simulink model "innerControllerTuning3"  (R2018a)
settings: Solver=VariableStepAuto  StartTime=0.0  StopTime=60  RelTol=1e-3
values from neighbouring files (symbols this model uses):
  d = 2.4*10^-3    (= 0.0024)    [innerInit.m]    (also in outerInit.m)
  dx0 = 0    [innerInit.m]
  dy0 = 0    [innerInit.m]
  dz0 = 0    [innerInit.m]
  g = 9.81    [innerInit.m]    (also in outerInit.m)
  Ixx = 5.9*10-3    (= 56)    [innerInit.m]    (also in outerInit.m = 0.0059)
  Iyy = 5.9*10-3    (= 56)    [innerInit.m]    (also in outerInit.m = 0.0059)
  Izz = 1.16*10-3    (= 8.6)    [innerInit.m]    (also in outerInit.m = 0.00116)
  K_lin = [   15.6000,    0.0000,    7.9000,    0.0000,         0 ... (first row only)    [innerInit.m]
  kr = 0.1    [innerInit.m]    (also in outerInit.m)
  kt = 0.1    [innerInit.m]    (also in outerInit.m)
  l = 0.255    [innerInit.m]    (also in outerInit.m)
  m = 0.5    [innerInit.m]    (also in outerInit.m)
  p0 = 0.5    [innerInit.m]
  phi0 = pi/4    (= 0.785398163397)    [innerInit.m]
  psi0 = pi/4    (= 0.785398163397)    [innerInit.m]
  q0 = 0.5    [innerInit.m]
  r0 = 2.7    [innerInit.m]
  theta0 = pi/4    (= 0.785398163397)    [innerInit.m]
  x0 = 1    [innerInit.m]    (also in outerInit.m = 2)
  y0 = 1    [innerInit.m]    (also in outerInit.m = 3)
  z0 = 0    [innerInit.m]    (also in outerInit.m = 4)
libraries: aerolibutil x1
settings Model: Creator=giuseppe  LastModifiedBy=giuseppe

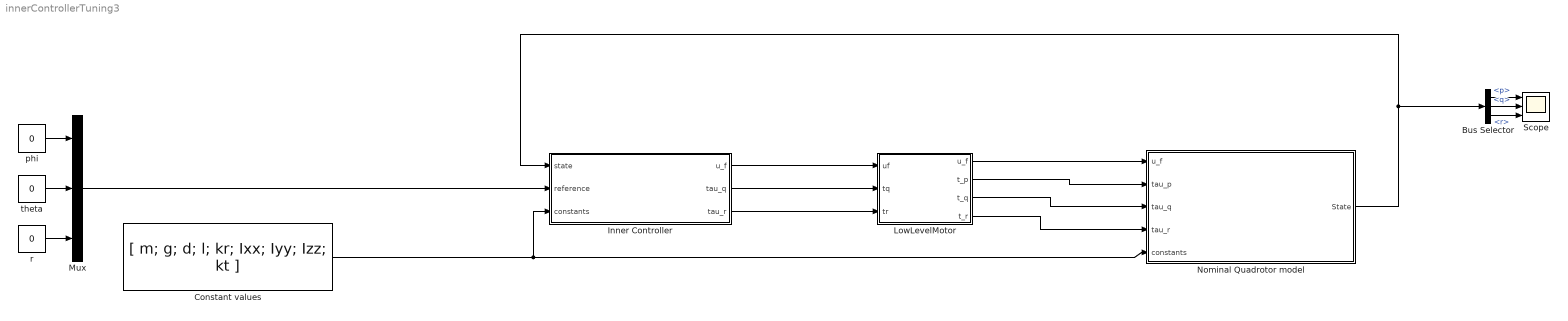
== system innerControllerTuning3 ==
  Bus Selector : BusSelector  OutputSignals=p,q,r
  Constant values : Constant  Value=[ m; g; d; l; kr; Ixx; Iyy; Izz; kt ]
  "Inner Controller " : Subsystem
  LowLevelMotor : Subsystem
  Mux : Mux  Inputs=3
  Nominal Quadrotor model : Subsystem
  Scope : Scope  NumInputPorts=3
  phi : Constant  Value=0
  r : Constant  Value=0
  theta : Constant  Value=0
  wires:
  LowLevelMotor/1(u_f) -> Nominal Quadrotor model/1(u_f)
  "Inner Controller "/2(tau_q) -> LowLevelMotor/2("tq ")
  LowLevelMotor/2(t_p) -> Nominal Quadrotor model/2(tau_p)
  "Inner Controller "/3(tau_r) -> LowLevelMotor/3(tr)
  "Inner Controller "/1(u_f) -> LowLevelMotor/1(uf)
  LowLevelMotor/3(t_q) -> Nominal Quadrotor model/3(tau_q)
  LowLevelMotor/4(t_r) -> Nominal Quadrotor model/4(tau_r)
  Constant values/1 -> "Inner Controller "/3(constants), Nominal Quadrotor model/5(constants)
  Nominal Quadrotor model/1(State) -> Bus Selector/1, "Inner Controller "/1(state)
  Mux/1 -> "Inner Controller "/2(reference)
  phi/1 -> Mux/1
  theta/1 -> Mux/2
  r/1 -> Mux/3
  Bus Selector/1 -> Scope/1  "<p>"
  Bus Selector/2 -> Scope/2  "<q>"
  Bus Selector/3 -> Scope/3  "<r>"

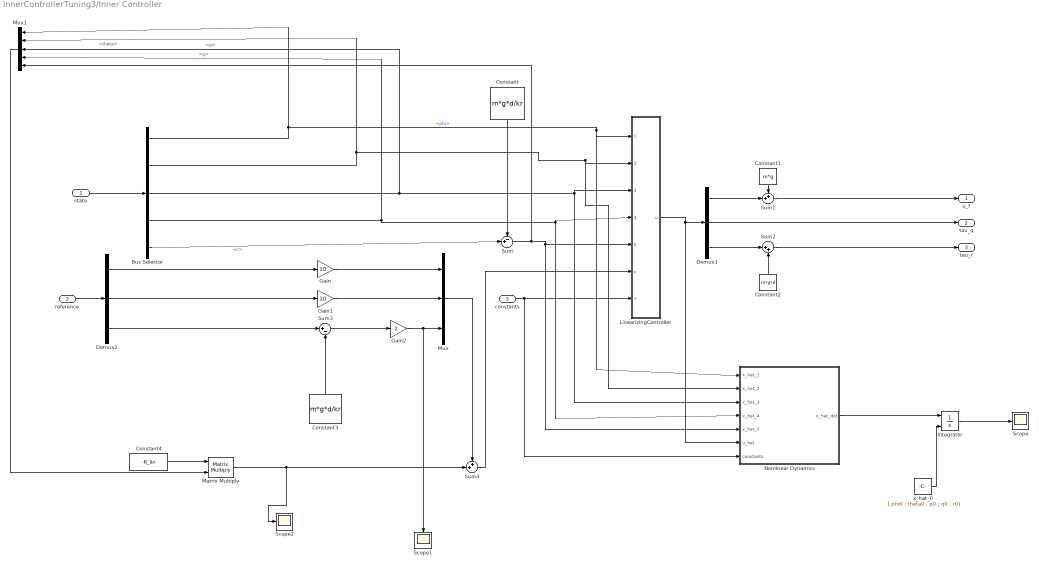
== system innerControllerTuning3/Inner Controller  ==
  state : Inport
  reference : Inport  Port=2
  constants : Inport  Port=3
  Bus Selector : BusSelector  OutputSignals=phi,theta,p,q,r
  Constant : Constant  Value=m*g*d/kr
  Constant1 : Constant  Value=m*g
  Constant2 : Constant  Value=m*g*d
  Constant3 : Constant  Value=m*g*d/kr
  Constant4 : Constant  Value=-K_lin
  Demux1 : Demux  Outputs=3
  Demux2 : Demux  Outputs=3
  Gain : Gain  Gain=10
  Gain1 : Gain  Gain=10
  Gain2 : Gain  Gain=2
  Integrator : Integrator  InitialConditionSource=external
  LinearizingController : MATLAB Function  TreatAsAtomicUnit=on
  Matrix Multiply : Product  Multiplication=Matrix(*)
  Mux : Mux  Inputs=3
  Mux1 : Mux  Inputs=5
  "Nonlinear Dynamics " : MATLAB Function  TreatAsAtomicUnit=on
  Scope : Scope
  Scope1 : Scope
  Scope2 : Scope
  Sum : Sum  Inputs=-+|
  Sum1 : Sum  Inputs=++|
  Sum2 : Sum  Inputs=|++
  Sum3 : Sum  Inputs=|+-
  Sum4 : Sum  Inputs=++|
  x_hat_0 : Constant  Value=[ phi0 ; theta0 ; p0 ; q0 ; r0]
  u_f : Outport
  tau_q : Outport  Port=2
  tau_r : Outport  Port=3
  wires:
  state/1 -> Bus Selector/1
  Bus Selector/3 -> Mux1/3, "Nonlinear Dynamics "/3(x_hat_3), LinearizingController/3(x3_hat)  "<p>"
  Bus Selector/4 -> Mux1/4, "Nonlinear Dynamics "/4(x_hat_4), LinearizingController/4(x4_hat)  "<q>"
  "Nonlinear Dynamics "/1(x_hat_dot) -> Integrator/1
  x_hat_0/1 -> Integrator/2
  Constant/1 -> Sum/1
  Sum/1 -> Mux1/5, "Nonlinear Dynamics "/5(x_hat_5), LinearizingController/5(x5_hat)
  Demux1/3 -> Sum2/1
  Demux1/1 -> Sum1/2
  Constant1/1 -> Sum1/1
  Sum1/1 -> u_f/1
  Demux1/2 -> tau_q/1
  Constant2/1 -> Sum2/2
  Sum2/1 -> tau_r/1
  LinearizingController/1(u) -> "Nonlinear Dynamics "/6(u_hat), Demux1/1
  constants/1 -> "Nonlinear Dynamics "/7(constants), LinearizingController/7(constants)
  Bus Selector/5 -> Sum/2  "<r>"
  reference/1 -> Demux2/1
  Constant3/1 -> Sum3/2
  Sum3/1 -> Gain2/1
  Bus Selector/1 -> Mux1/1, "Nonlinear Dynamics "/1(x_hat_1), LinearizingController/1(x1_hat)  "<phi>"
  Bus Selector/2 -> Mux1/2, "Nonlinear Dynamics "/2(x_hat_2), LinearizingController/2(x2_hat)  "<theta>"
  Demux2/1 -> Gain/1
  Demux2/2 -> Gain1/1
  Constant4/1 -> Matrix Multiply/1
  Mux1/1 -> Matrix Multiply/2
  Mux/1 -> Sum4/1
  Sum4/1 -> LinearizingController/6(v)
  Gain/1 -> Mux/1
  Gain1/1 -> Mux/2
  Demux2/3 -> Sum3/1
  Gain2/1 -> Mux/3, Scope1/1
  Matrix Multiply/1 -> Scope2/1, Sum4/2
  Integrator/1 -> Scope/1

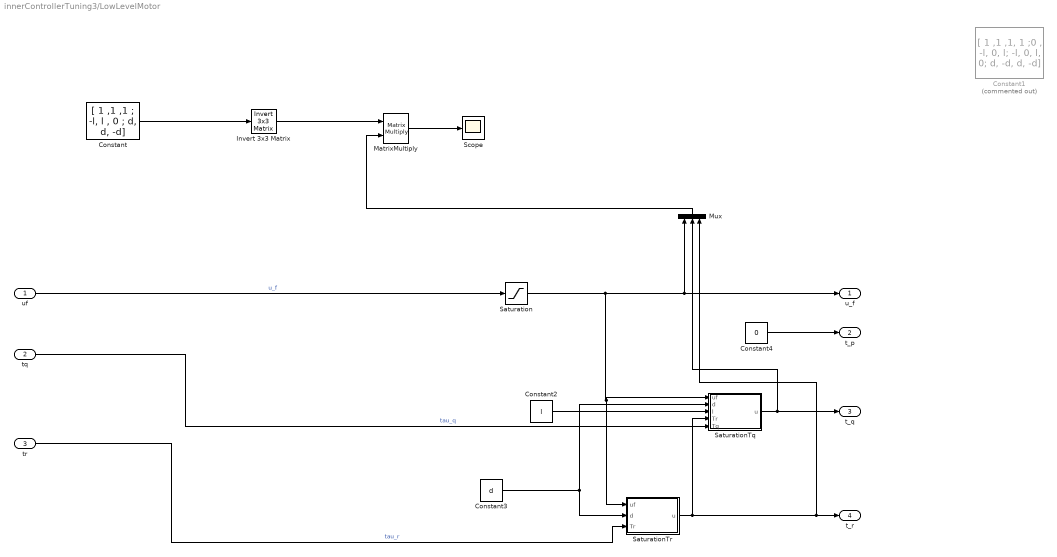
== system innerControllerTuning3/LowLevelMotor ==
  uf : Inport
  "tq " : Inport  Port=2
  tr : Inport  Port=3
  Constant : Constant  Value=[ 1 ,1 ,1 ; -l, l , 0 ; d, d, -d]
  Constant1 : Constant  Commented=on  Value="[ 1 ,1 ,1, 1 ;0 , -l, 0, l;  -l, 0, l, 0; d, -d, d, -d]"
  Constant2 : Constant  Value=l
  Constant3 : Constant  Value=d
  Constant4 : Constant  Value=0
  Invert 3x3 Matrix : aerolibutil/Invert  3x3 Matrix
  MatrixMultiply : Product  Multiplication=Matrix(*)
  Mux : Mux  Inputs=3
  Saturation : Saturate  UpperLimit=30
  SaturationTq : MATLAB Function  TreatAsAtomicUnit=on
  SaturationTr : MATLAB Function  TreatAsAtomicUnit=on
  Scope : Scope
  u_f : Outport
  t_p : Outport  Port=2
  t_q : Outport  Port=3
  t_r : Outport  Port=4
  wires:
  "tq "/1 -> SaturationTq/5(Tq)  "tau_q"
  tr/1 -> SaturationTr/3(Tr)  "tau_r"
  uf/1 -> Saturation/1  "u_f"
  Constant/1 -> Invert 3x3 Matrix/1
  Constant4/1 -> t_p/1
  Constant3/1 -> SaturationTq/2(d), SaturationTr/2(d)
  SaturationTr/1(u) -> SaturationTq/4(Tr), Mux/3, t_r/1
  SaturationTq/1(u) -> Mux/2, t_q/1
  Invert 3x3 Matrix/1 -> MatrixMultiply/1
  Saturation/1 -> SaturationTr/1(uf), SaturationTq/1(uf), u_f/1, Mux/1
  MatrixMultiply/1 -> Scope/1
  Constant2/1 -> SaturationTq/3(l)
  Mux/1 -> MatrixMultiply/2

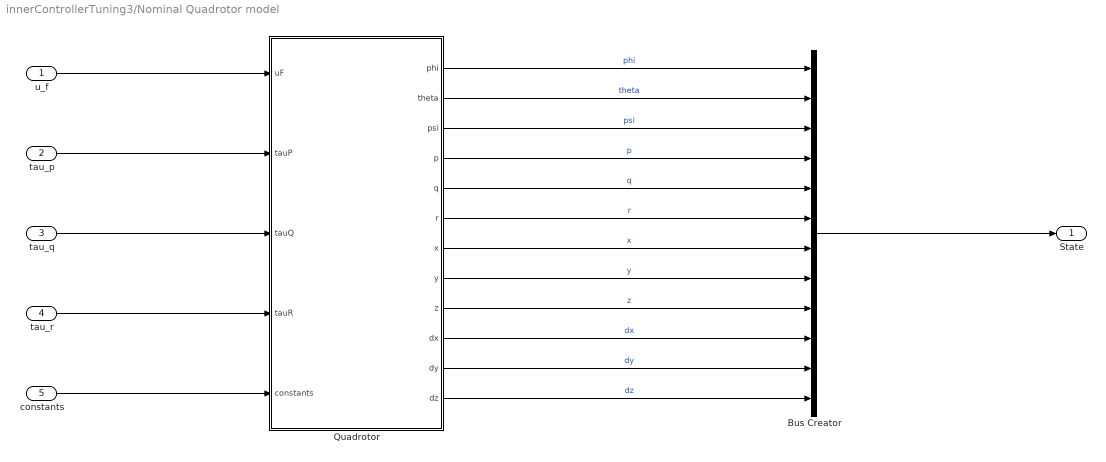
== system innerControllerTuning3/Nominal Quadrotor model ==
  u_f : Inport
  tau_p : Inport  Port=2
  tau_q : Inport  Port=3
  tau_r : Inport  Port=4
  constants : Inport  Port=5
  Bus Creator : BusCreator  Inputs=12
  "Quadrotor " : Subsystem
  State : Outport
  wires:
  u_f/1 -> "Quadrotor "/1(uF)
  tau_q/1 -> "Quadrotor "/3(tauQ)
  tau_r/1 -> "Quadrotor "/4(tauR)
  constants/1 -> "Quadrotor "/5(constants)
  tau_p/1 -> "Quadrotor "/2(tauP)
  "Quadrotor "/1(phi) -> Bus Creator/1  "phi"
  "Quadrotor "/2(theta) -> Bus Creator/2  "theta"
  "Quadrotor "/3(psi) -> Bus Creator/3  "psi"
  "Quadrotor "/4(p) -> Bus Creator/4  "p"
  "Quadrotor "/5(q) -> Bus Creator/5  "q"
  "Quadrotor "/6(r) -> Bus Creator/6  "r"
  "Quadrotor "/7(x) -> Bus Creator/7  "x"
  "Quadrotor "/8(y) -> Bus Creator/8  "y"
  "Quadrotor "/9(z) -> Bus Creator/9  "z"
  Bus Creator/1 -> State/1
  "Quadrotor "/10(dx) -> Bus Creator/10  "dx"
  "Quadrotor "/11(dy) -> Bus Creator/11  "dy"
  "Quadrotor "/12(dz) -> Bus Creator/12  "dz"

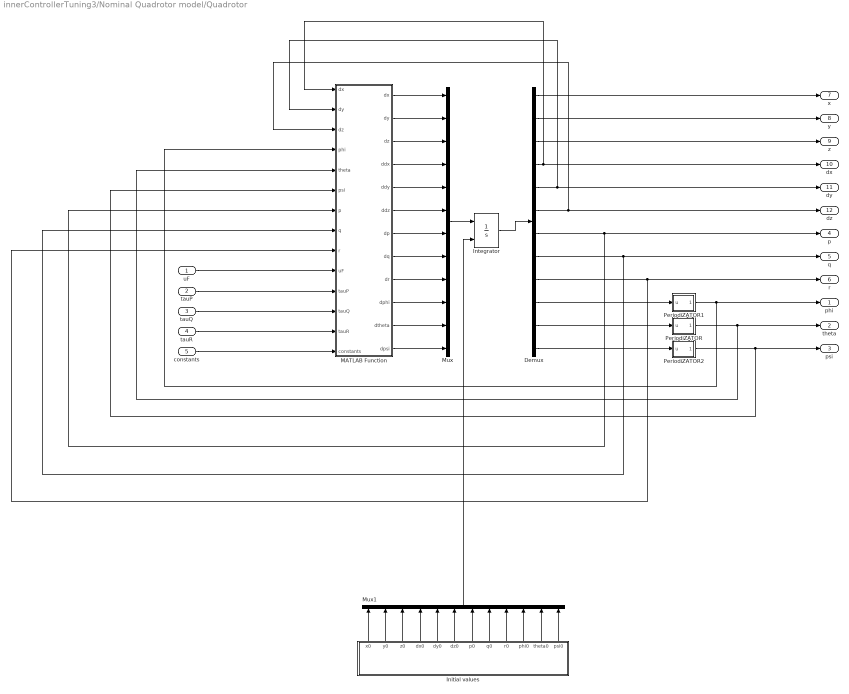
== system innerControllerTuning3/Nominal Quadrotor model/Quadrotor  ==
  uF : Inport
  tauP : Inport  Port=2
  tauQ : Inport  Port=3
  tauR : Inport  Port=4
  constants : Inport  Port=5
  Demux : Demux  Outputs=12
  "Initial values " : Subsystem
  Integrator : Integrator  InitialConditionSource=external
  MATLAB Function : MATLAB Function  TreatAsAtomicUnit=on
  Mux : Mux  Inputs=12
  Mux1 : Mux  Inputs=12
  PeriodiZATOR : MATLAB Function  TreatAsAtomicUnit=on
  PeriodiZATOR1 : MATLAB Function  TreatAsAtomicUnit=on
  PeriodiZATOR2 : MATLAB Function  TreatAsAtomicUnit=on
  phi : Outport
  theta : Outport  Port=2
  psi : Outport  Port=3
  p : Outport  Port=4
  q : Outport  Port=5
  r : Outport  Port=6
  x : Outport  Port=7
  y : Outport  Port=8
  z : Outport  Port=9
  dx : Outport  Port=10
  dy : Outport  Port=11
  dz : Outport  Port=12
  wires:
  uF/1 -> MATLAB Function/10(uF)
  tauP/1 -> MATLAB Function/11(tauP)
  tauQ/1 -> MATLAB Function/12(tauQ)
  tauR/1 -> MATLAB Function/13(tauR)
  PeriodiZATOR/1(angle) -> MATLAB Function/5(theta), theta/1
  PeriodiZATOR1/1(angle) -> MATLAB Function/4(phi), phi/1
  PeriodiZATOR2/1(angle) -> MATLAB Function/6(psi), psi/1
  constants/1 -> MATLAB Function/14(constants)
  MATLAB Function/1(dx) -> Mux/1
  MATLAB Function/2(dy) -> Mux/2
  MATLAB Function/3(dz) -> Mux/3
  MATLAB Function/4(ddx) -> Mux/4
  MATLAB Function/5(ddy) -> Mux/5
  MATLAB Function/6(ddz) -> Mux/6
  MATLAB Function/10(dphi) -> Mux/10
  MATLAB Function/11(dtheta) -> Mux/11
  MATLAB Function/12(dpsi) -> Mux/12
  Mux/1 -> Integrator/1
  "Initial values "/1(x0) -> Mux1/1
  "Initial values "/2(y0) -> Mux1/2
  "Initial values "/3(z0) -> Mux1/3
  "Initial values "/4(dx0) -> Mux1/4
  "Initial values "/5(dy0) -> Mux1/5
  "Initial values "/6(dz0) -> Mux1/6
  "Initial values "/7(p0) -> Mux1/7
  "Initial values "/8(q0) -> Mux1/8
  "Initial values "/9(r0) -> Mux1/9
  "Initial values "/10(phi0) -> Mux1/10
  "Initial values "/11(theta0) -> Mux1/11
  "Initial values "/12(psi0) -> Mux1/12
  Mux1/1 -> Integrator/2
  Integrator/1 -> Demux/1
  Demux/1 -> x/1
  Demux/2 -> y/1
  Demux/3 -> z/1
  Demux/5 -> dy/1, MATLAB Function/2("dy ")
  Demux/6 -> dz/1, MATLAB Function/3("dz ")
  Demux/10 -> PeriodiZATOR1/1(u)
  Demux/11 -> PeriodiZATOR/1(u)
  Demux/12 -> PeriodiZATOR2/1(u)
  Demux/9 -> r/1, MATLAB Function/9(r)
  MATLAB Function/7(dp) -> Mux/7
  MATLAB Function/8(dq) -> Mux/8
  Demux/7 -> p/1, MATLAB Function/7(p)
  Demux/8 -> q/1, MATLAB Function/8(q)
  MATLAB Function/9(dr) -> Mux/9
  Demux/4 -> dx/1, MATLAB Function/1("dx ")

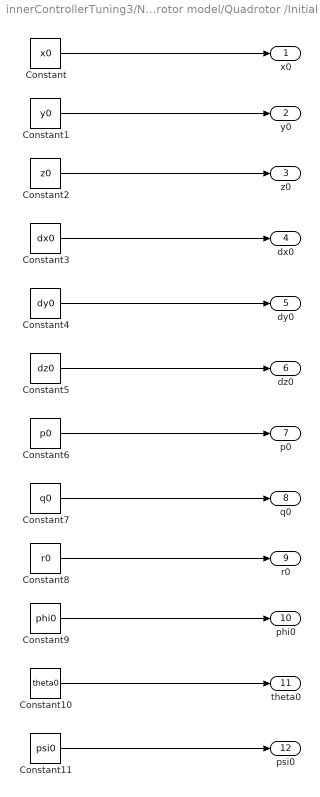
== system innerControllerTuning3/Nominal Quadrotor model/Quadrotor /Initial values  ==
  Constant : Constant  Value=x0
  Constant1 : Constant  Value=y0
  Constant10 : Constant  Value=theta0
  Constant11 : Constant  Value=psi0
  Constant2 : Constant  Value=z0
  Constant3 : Constant  Value=dx0
  Constant4 : Constant  Value=dy0
  Constant5 : Constant  Value=dz0
  Constant6 : Constant  Value=p0
  Constant7 : Constant  Value=q0
  Constant8 : Constant  Value=r0
  Constant9 : Constant  Value=phi0
  x0 : Outport
  y0 : Outport  Port=2
  z0 : Outport  Port=3
  dx0 : Outport  Port=4
  dy0 : Outport  Port=5
  dz0 : Outport  Port=6
  p0 : Outport  Port=7
  q0 : Outport  Port=8
  r0 : Outport  Port=9
  phi0 : Outport  Port=10
  theta0 : Outport  Port=11
  psi0 : Outport  Port=12
  wires:
  Constant/1 -> x0/1
  Constant1/1 -> y0/1
  Constant2/1 -> z0/1
  Constant3/1 -> dx0/1
  Constant4/1 -> dy0/1
  Constant5/1 -> dz0/1
  Constant6/1 -> p0/1
  Constant7/1 -> q0/1
  Constant8/1 -> r0/1
  Constant9/1 -> phi0/1
  Constant10/1 -> theta0/1
  Constant11/1 -> psi0/1

== matlab function innerControllerTuning3/Inner Controller /LinearizingController ==
  data: x1_hat input; u output; x2_hat input; x3_hat input; x4_hat input; x5_hat input; v input; constants input
function u = fcn(x1_hat,x2_hat,x3_hat,x4_hat,x5_hat, v, constants)

m= constants(1,1);
g= constants(2,1);
d= constants(3,1);
l= constants(4,1);
kr= constants(5,1);
Ixx= constants(6,1);
Iyy= constants(7,1);
Izz= constants(8,1);

alfa = zeros(3,1);

%% Non-robust feedback-linearation

alfa(1,1) = (2*Ixx*((kr*x3_hat - x4_hat*(x5_hat + (d*g*m)/kr)*(Ixx - Izz))/Ixx + (sin(x1_hat)*tan(x2_hat)*(x5_hat + (d*g*m)/kr) - x4_hat*cos(x1_hat)*tan(x2_hat))*(x3_hat + cos(x1_hat)*tan(x2_hat)*(x5_hat + (d*g*m)/kr) + x4_hat*sin(x1_hat)*tan(x2_hat)) + (sin(x1_hat)*(x5_hat + (d*g*m)/kr) - x4_hat*cos(x1_hat))*(cos(x1_hat)*(x5_hat + (d*g*m)/kr)*(tan(x2_hat)^2 + 1) + x4_hat*sin(x1_hat)*(tan(x2_hat)^2 + 1)) + (sin(x1_hat)*tan(x2_hat)*(kr*x4_hat + x3_hat*(x5_hat + (d*g*m)/kr)*(Ixx - Izz)))/Ixx + (kr*x5_hat*cos(x1_hat)*tan(x2_hat))/Izz))/l - (2*Ixx*sin(x1_hat)*tan(x2_hat)*((cos(x1_hat)*(x5_hat + (d*g*m)/kr) + x4_hat*sin(x1_hat))*(x3_hat + cos(x1_hat)*tan(x2_hat)*(x5_hat + (d*g*m)/kr) + x4_hat*sin(x1_hat)*tan(x2_hat)) + (cos(x1_hat)*(kr*x4_hat + x3_hat*(x5_hat + (d*g*m)/kr)*(Ixx - Izz)))/Ixx - (kr*x5_hat*sin(x1_hat))/Izz))/(l*cos(x1_hat)) - (kr*x5_hat*(2*Ixx*d*cos(x1_hat)^2*tan(x2_hat) - Izz*l*cos(x1_hat) + 2*Ixx*d*sin(x1_hat)^2*tan(x2_hat)))/(Izz*d*l*cos(x1_hat));
alfa(2,1) = (Ixx*((cos(x1_hat)*(x5_hat + (d*g*m)/kr) + x4_hat*sin(x1_hat))*(x3_hat + cos(x1_hat)*tan(x2_hat)*(x5_hat + (d*g*m)/kr) + x4_hat*sin(x1_hat)*tan(x2_hat)) + (cos(x1_hat)*(kr*x4_hat + x3_hat*(x5_hat + (d*g*m)/kr)*(Ixx - Izz)))/Ixx - (kr*x5_hat*sin(x1_hat))/Izz))/cos(x1_hat) + (Ixx*kr*x5_hat*sin(x1_hat))/(Izz*cos(x1_hat));
alfa(3,1) = kr*x5_hat;


beta =  [
         (2*Ixx)/l, -(2*Ixx*sin(x1_hat)*sin(x2_hat))/(l*cos(x1_hat)*cos(x2_hat)), -(2*Ixx*d*sin(x2_hat)-Izz*l*cos(x1_hat)*cos(x2_hat))/(d*l*cos(x1_hat)*cos(x2_hat));
         0,                                              Ixx/cos(x1_hat),                                                        (Ixx*sin(x1_hat))/cos(x1_hat);
         0,                                                            0,                                                                                  Izz];

%% Robust feedback linearization

% alfa(1,1) = x1_hat*((d*g*m*((2*Ixx*((d*g*m)/kr + (d*g*m*(Ixx - Izz))/(Ixx*kr)))/l + (2*kr*sin(x1_hat)*tan(x2_hat))/(l*cos(x1_hat))))/kr - (2*Ixx*d^2*g^2*m^2)/(kr^2*l)) - (sin(x1_hat)*(x5_hat + (d*g*m)/kr) - x4_hat*cos(x1_hat))*((2*Ixx*((d*g*m)/kr + (d*g*m*(Ixx - Izz))/(Ixx*kr)))/l + (2*kr*sin(x1_hat)*tan(x2_hat))/(l*cos(x1_hat))) + x2_hat*((d*g*m*((2*kr)/l - (2*Ixx*sin(x1_hat)*tan(x2_hat)*((d*g*m)/kr + (d*g*m*(Ixx - Izz))/(Ixx*kr)))/(l*cos(x1_hat))))/kr + (2*Ixx*d^2*g^2*m^2*sin(x1_hat)*tan(x2_hat))/(kr^2*l*cos(x1_hat))) - ((2*kr)/l - (2*Ixx*sin(x1_hat)*tan(x2_hat)*((d*g*m)/kr + (d*g*m*(Ixx - Izz))/(Ixx*kr)))/(l*cos(x1_hat)))*(x3_hat + cos(x1_hat)*tan(x2_hat)*(x5_hat + (d*g*m)/kr) + x4_hat*sin(x1_hat)*tan(x2_hat)) + (2*Ixx*((kr*x3_hat - x4_hat*(x5_hat + (d*g*m)/kr)*(Ixx - Izz))/Ixx + (sin(x1_hat)*tan(x2_hat)*(x5_hat + (d*g*m)/kr) - x4_hat*cos(x1_hat)*tan(x2_hat))*(x3_hat + cos(x1_hat)*tan(x2_hat)*(x5_hat + (d*g*m)/kr) + x4_hat*sin(x1_hat)*tan(x2_hat)) + (sin(x1_hat)*(x5_hat + (d*g*m)/kr) - x4_hat*cos(x1_hat))*(cos(x1_hat)*(x5_hat + (d*g*m)/kr)*(tan(x2_hat)^2 + 1) + x4_hat*sin(x1_hat)*(tan(x2_hat)^2 + 1)) + (sin(x1_hat)*tan(x2_hat)*(kr*x4_hat + x3_hat*(x5_hat + (d*g*m)/kr)*(Ixx - Izz)))/Ixx + (kr*x5_hat*cos(x1_hat)*tan(x2_hat))/Izz))/l - (2*Ixx*sin(x1_hat)*tan(x2_hat)*((cos(x1_hat)*(x5_hat + (d*g*m)/kr) + x4_hat*sin(x1_hat))*(x3_hat + cos(x1_hat)*tan(x2_hat)*(x5_hat + (d*g*m)/kr) + x4_hat*sin(x1_hat)*tan(x2_hat)) + (cos(x1_hat)*(kr*x4_hat + x3_hat*(x5_hat + (d*g*m)/kr)*(Ixx - Izz)))/Ixx - (kr*x5_hat*sin(x1_hat))/Izz))/(l*cos(x1_hat));
% alfa(2,1) = (kr*x5_hat*sin(x1_hat) - kr*x4_hat*cos(x1_hat) + d*g*m*sin(x1_hat))/cos(x1_hat) + (Ixx*((cos(x1_hat)*(kr*x4_hat + (x3_hat*(kr*x5_hat + d*g*m)*(Ixx - Izz))/kr))/Ixx + ((kr*x5_hat*cos(x1_hat) + kr*x4_hat*sin(x1_hat) + d*g*m*cos(x1_hat))*(x3_hat + x4_hat*sin(x1_hat)*tan(x2_hat) + (cos(x1_hat)*tan(x2_hat)*(kr*x5_hat + d*g*m))/kr))/kr - (kr*x5_hat*sin(x1_hat))/Izz))/cos(x1_hat) - (d*g*m*x1_hat)/cos(x1_hat) - (d*g*m*(2*Ixx - Izz)*(x3_hat + x4_hat*sin(x1_hat)*tan(x2_hat) + (cos(x1_hat)*tan(x2_hat)*(kr*x5_hat + d*g*m))/kr))/(kr*cos(x1_hat)) + (d^2*g^2*m^2*x2_hat*(Ixx - Izz))/(kr^2*cos(x1_hat));
% alfa(3,1) = 0;
% 
% beta = [
%         1, -(2*sin(x1_hat)*sin(x2_hat))/(l*cos(x1_hat)*cos(x2_hat)), -(2*Ixx*sin(x2_hat))/(Izz*l*cos(x1_hat)*cos(x2_hat));
%         0,                                            1/cos(x1_hat),                  (Ixx*sin(x1_hat))/(Izz*cos(x1_hat));
%         0,                                                        0,                                                    1];
    
u = alfa + beta*v;

== matlab function innerControllerTuning3/LowLevelMotor/SaturationTr ==
  data: uf input; u output; d input; Tr input
function u = fcn(uf, d, Tr)

if abs(Tr) > d*uf
    Tr = sign(Tr)*d*uf;
end

u = Tr;

== matlab function innerControllerTuning3/Inner Controller /Nonlinear Dynamics  ==
  data: x_hat_1 input; x_hat_2 input; x_hat_3 input; x_hat_4 input; x_hat_5 input; x_hat_dot output; u_hat input; constants input
function x_hat_dot = fcn(x_hat_1,x_hat_2,x_hat_3,x_hat_4,x_hat_5,u_hat,constants)

m= constants(1,1);
g= constants(2,1);
d= constants(3,1);
l= constants(4,1);
kr= constants(5,1);
Ixx= constants(6,1);
Iyy= constants(7,1);
Izz= constants(8,1);

x_hat = [x_hat_1;
        x_hat_2;
        x_hat_3;
        x_hat_4;
        x_hat_5];

f = [
    x_hat(3,1)+x_hat(4,1)*sin(x_hat(1,1))*tan(x_hat(2,1)) + ( x_hat(5,1)+ m*g*d/kr)*cos(x_hat(1,1))*tan(x_hat(2,1));
    x_hat(4,1)*cos(x_hat(1,1))- (x_hat(5,1)+ m*g*d/kr)*sin(x_hat(1,1)) ;
    1/Ixx*( -kr*x_hat(3,1)- x_hat(4,1)*(x_hat(5,1)+ m*g*d/kr)*(Izz - Ixx));
    1/Iyy*( -kr*x_hat(4,1)- x_hat(3,1)*(x_hat(5,1)+ m*g*d/kr)*(Ixx - Izz));
    1/Izz*(-kr* x_hat(5,1));    
    ];
G = [
    0 , 0 , 0;
    0,  0 , 0;
    l/(2*Ixx), 0 , -l/(2*d*Ixx)
    0,  1/Iyy  , 0 ;
    0 ,  0   ,  1/Izz;
    ];

    
x_hat_dot = f + G*u_hat;

== matlab function innerControllerTuning3/LowLevelMotor/SaturationTq ==
  data: uf input; u output; d input; l input; Tr input; Tq input
function u = fcn(uf, d, l, Tr, Tq)

if abs(Tq) > (0.5*l*(uf+Tr/d))
    Tq = sign(Tq)*(0.5*l*(uf+Tr/d));
end

u = Tq;

== matlab function innerControllerTuning3/Nominal Quadrotor model/Quadrotor /MATLAB Function ==
  data: dx output; dy output; dz output; dx input; dy input; dz input; phi input; theta input; psi input; p input; q input; r input; uF input; ddx output; tauP input; tauQ input; tauR input; ddy output; ddz output; dp output; dq output; dr output; dphi output; dtheta output; dpsi output; constants input
function [dx,dy,dz,ddx,ddy,ddz,dp,dq,dr,dphi,dtheta,dpsi] = fcn(dx, dy, dz, phi, theta, psi, p, q, r, uF, tauP, tauQ, tauR, constants)

    m= constants(1,1);
    g= constants(2,1);
    d= constants(3,1);
    l= constants(4,1);
    kr= constants(5,1);
    Ixx= constants(6,1);
    Iyy= constants(7,1);
    Izz= constants(8,1);
    kt = constants(9,1);

    
    ddx = (1/m)*((cos(phi)*cos(psi)*sin(theta) + sin(phi)*sin(psi))*uF - kt*dx);
    
    ddy = (1/m)*((cos(phi)*sin(theta)*sin(psi) - cos(psi)*sin(phi))*uF - kt*dy);
    
    ddz = (1/m)*((cos(theta)*cos(phi))*uF - m*g - kt*dz);
    
%     dp = (1/Ixx)*(-kr*p - q*r*(Izz - Iyy) + tauP);

    dp = (1/Ixx)*(-kr*p - q*r*(Izz - Iyy) + l/2*(uF - tauR/d));
    
    dq = (1/Iyy)*(-kr*q - p*r*(Ixx - Izz) + tauQ);
    
    dr = (1/Izz)*(-kr*r - p*q*(Iyy - Ixx) + tauR);
    
%     dr = 1/Izz*(-kr*r + tauR);
    
    dphi = p + q*sin(phi)*tan(theta) + r*cos(phi)*tan(theta);
    
    dtheta = q*cos(phi) - r*sin(phi);
    
    dpsi = (1/cos(theta))*(q*sin(phi) + r*cos(phi));

== matlab function innerControllerTuning3/Nominal Quadrotor model/Quadrotor /PeriodiZATOR ==
  data: u input; angle output
function angle = fcn(u)

y = sin(u);
x = cos(u);

% angle = mod(u, 2*pi)
angle = atan2(y,x);

== matlab function innerControllerTuning3/Nominal Quadrotor model/Quadrotor /PeriodiZATOR1 ==
  data: u input; angle output
function angle = fcn(u)

y = sin(u);
x = cos(u);

% angle = mod(u, 2*pi)
angle = atan2(y,x);

== matlab function innerControllerTuning3/Nominal Quadrotor model/Quadrotor /PeriodiZATOR2 ==
  data: u input; angle output
function angle = fcn(u)

y = sin(u);
x = cos(u);

% angle = mod(u, 2*pi);
angle = atan2(y,x);
